simulink model "Snap"  (R2020a)
settings: Solver=FixedStepAuto  StartTime=0.0  StopTime=10.0  FixedStep=0.1  MaxStep=0.1  RelTol=1e-3
model workspace (MAT data in the model file):
  midSnapParamTop = Simulink.Parameter
  midSnapParamTop.Value = 3
  midSnapParamTop.DataType = 'int32'
  midSnapParamTop.Dimensions = [1 1]
  paramDouble = Simulink.Parameter
  paramDouble.Value = 6
  paramDouble.DataType = 'auto'
  paramDouble.Dimensions = [1 1]
  paramInt = Simulink.Parameter
  paramInt.Value = 4
  paramInt.DataType = 'int32'
  paramInt.Dimensions = [1 1]
settings Model: DataDictionary=TestConfig.sldd  TunableVars=param  TunableVarsStorageClass=Auto  ParameterArgumentNames=midSnapParamTop,paramInt  OrderedModelArguments=off  Creator=raarenst  LastModifiedBy=toma
settings OptimizationCC: DefaultParameterBehavior=Inlined  EnhancedBackFolding=on  PassReuseOutputArgsAs=Individual arguments  ZeroExternalMemoryAtStartup=off  ZeroInternalMemoryAtStartup=off  OptimizeBlockOrder=speed  DifferentSizesBufferReuse=on  OptimizationCustomize=off  EfficientTunableParamExpr=on
settings DebuggingCC: UnderspecifiedInitializationDetection=Classic  MergeDetectMultiDrivingBlocksExec=none  ParameterTunabilityLossMsg=error  ModelReferenceSymbolNameMessage=none
settings ModelReferenceCC: PropagateSignalLabelsOutOfModel=off
settings SFSimCC: MATLABDynamicMemAlloc=off
settings RTWCC: Description=CIGRE export target  SystemTargetFile=cigre.tlc  TemplateMakefile=cigre_tmf  Toolchain=CIGRE DLL - Microsoft Visual C++ 2019 (64bit) | nmake makefile (64-bit Windows)
settings CodeAppCC: ForceParamTrailComments=on  IgnoreCustomStorageClasses=off  OperatorAnnotations=on  SimulinkDataObjDesc=on  SFDataObjDesc=on  InsertBlockDesc=on
settings STFCustomTargetCC: TargetLangStandard=C99 (ISO)  MultiwordLength=256  GenerateSampleERTMain=on  CompOptLevelCompliant=on  CombineOutputUpdateFcns=on  ERTCustomFileBanners=on  MultiInstanceERTCode=on  CodeInterfacePackaging=Reusable function  SupportContinuousTime=off  SupportNonInlinedSFcns=off  RemoveResetFunc=on  MATLABClassNameForMDSCustomization=Simulink.SoftwareTarget.ERTCustomization  UseToolchainInfoCompliant=on  SystemTargetFile=cigre.tlc
settings ERTTargetCC: TargetLangStandard=C99 (ISO)  GenerateSampleERTMain=on  ParMdlRefBuildCompliant=off  ConcurrentExecutionCompliant=off  MultiInstanceERTCode=on  CodeInterfacePackaging=Reusable function  ModelStepFunctionPrototypeControlCompliant=off  CPPClassGenCompliant=off  InlinedParameterPlacement=NonHierarchical  RootIOFormat=Structure reference  ERTCustomFileTemplate=example_file_process.tlc

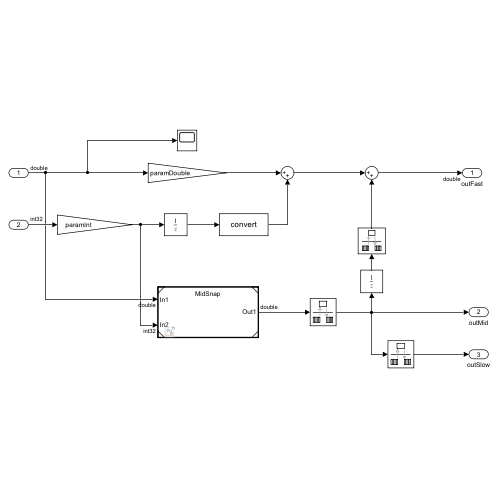
[thumbnail: Simulink's stored preview of the top-level diagram]
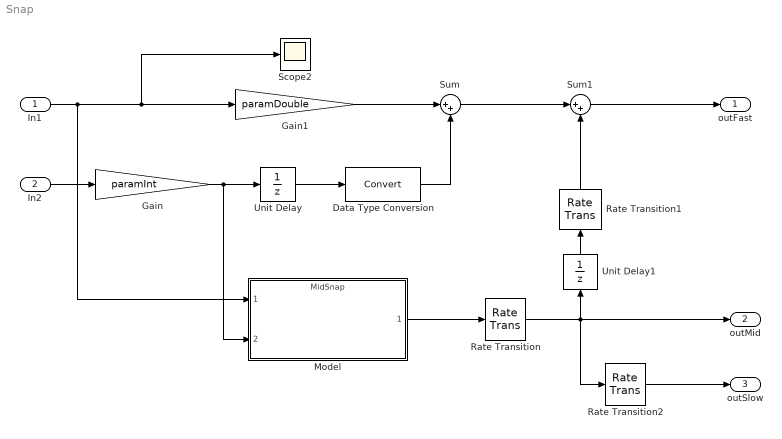
== system Snap ==
  In1 : Inport  OutDataTypeStr=double  SampleTime=0.1
  In2 : Inport  Port=2  OutDataTypeStr=int32  SampleTime=0.1
  Data Type Conversion : DataTypeConversion
  Gain : Gain  Gain=paramInt  ParamDataTypeStr=int32  OutDataTypeStr=int32
  Gain1 : Gain  Gain=paramDouble  ParamDataTypeStr=double  OutDataTypeStr=Inherit: Same as input
  Model : ModelReference  ModelNameDialog=MidSnap  ParameterArgumentNames=midSnapParam  ParameterArgumentValues=midSnapParamTop  UsingDefaultArgumentValue=0  SimulationMode=Normal  ModelReferenceVersion=1.4
  Rate Transition : RateTransition  OutPortSampleTime=0.5
  Rate Transition1 : RateTransition  OutPortSampleTime=0.1
  Rate Transition2 : RateTransition  OutPortSampleTime=1
  Scope2 : Scope
  Sum : Sum  Inputs=|++
  Sum1 : Sum  Inputs=|++
  Unit Delay : UnitDelay  InitialCondition=3  SampleTime=-1  HasFrameUpgradeWarning=on
  Unit Delay1 : UnitDelay  InitialCondition=3  SampleTime=-1  HasFrameUpgradeWarning=on
  outFast : Outport  OutDataTypeStr=double
  outMid : Outport  Port=2
  outSlow : Outport  Port=3
  wires:
  In2/1 -> Gain/1
  Gain/1 -> Model/2, Unit Delay/1
  Unit Delay/1 -> Data Type Conversion/1
  In1/1 -> Model/1, Scope2/1, Gain1/1
  Data Type Conversion/1 -> Sum/2
  Model/1 -> Rate Transition/1
  Sum1/1 -> outFast/1
  Gain1/1 -> Sum/1
  Sum/1 -> Sum1/1
  Rate Transition/1 -> Rate Transition2/1, Unit Delay1/1, outMid/1
  Rate Transition1/1 -> Sum1/2
  Unit Delay1/1 -> Rate Transition1/1
  Rate Transition2/1 -> outSlow/1
